simulink model "timu32_sim"  (R2021b)
settings: Solver=VariableStepAuto  StartTime=0.0  StopTime=10.0  RelTol=1e-3
settings Model: Creator=1412  LastModifiedBy=1412

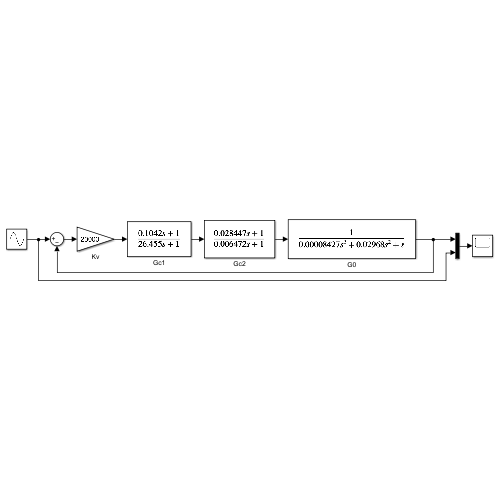
[thumbnail: Simulink's stored preview of the top-level diagram]
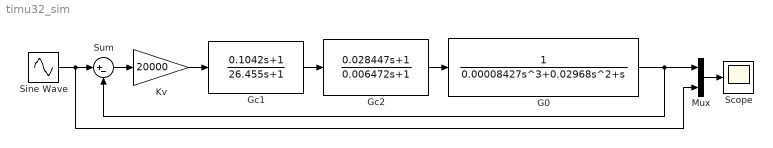
== system timu32_sim ==
  G0 : TransferFcn  Denominator=[0.00008427 0.02968 1 0]
  Gc1 : TransferFcn  Numerator=[0.1042 1]  Denominator=[26.455 1]
  Gc2 : TransferFcn  Numerator=[0.028447 1]  Denominator=[0.006472 1]
  Kv : Gain  Gain=20000
  Mux : Mux  Inputs=2
  Scope : Scope
  Sine Wave : Sin  Amplitude=666  Frequency=0.6  SampleTime=0
  Sum : Sum  Inputs=|+-
  wires:
  Sum/1 -> Kv/1
  Sine Wave/1 -> Mux/2, Sum/1
  Gc1/1 -> Gc2/1
  Gc2/1 -> G0/1
  G0/1 -> Sum/2, Mux/1
  Mux/1 -> Scope/1
  Kv/1 -> Gc1/1
